simulink model "Steering"  (R2017a)
settings: Solver=VariableStepAuto  StartTime=0.0  StopTime=10  FixedStep=0.05  RelTol=1e-3
values from neighbouring files (symbols this model uses):
  distance_of_CG = vehical_length/2    (= 0.1825)    [initialize.m]
  H = Center_G(1)    [initialize.m]
  K = Center_G(2)    [initialize.m]
  psi_init = deg2rad(60)    [initialize.m]
  test_case = 2    [initialize.m]
  x0 = 0    [initialize.m]
  x_init = 0    [initialize.m]
  y0 = 0    [initialize.m]
  y_init = 1    [initialize.m]
undefined symbols (not defined in the file): parabora_coefficient, Radius, Theta, vehical_length, x_intersept, y_intersept
libraries: simulink_extras x5, frdmtfcshieldlib x2, simulink x1
settings Model: SnapshotInterval=1  Creator=dell  LastModifiedBy=dell
settings DebuggingCC: InheritedTsInSrcMsg=error

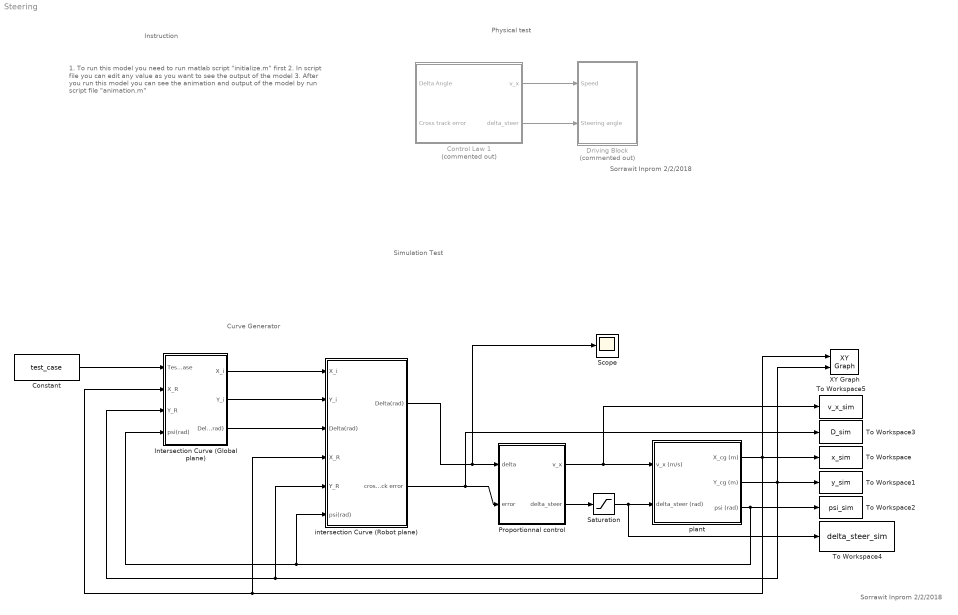
== system Steering ==
  note: Sorrawit Inprom
      | 2/2/2018
  note: Curve Generator
  note: Simulation Test
  note: Physical test
  note: Sorrawit Inprom
      | 2/2/2018
  note: Instruction
  note: 1. To run this model you need to run matlab script "initialize.m" first
      |
      | 2. In script file you can edit any value as you want to see the output of the model
      |
      | 3. After you run this model you can see the animation and output of the model by run script file "animation.m"
  Constant : Constant  Value=test_case
  Control Law 1 : Subsystem  Commented=on
  Driving Block : Subsystem  Commented=on
  Intersection Curve (Global plane) : Subsystem
  Proportionnal control : Subsystem
  Saturation : Saturate  UpperLimit=deg2rad(25)  LowerLimit=-deg2rad(25)
  Scope : Scope
  To Workspace : ToWorkspace  VariableName=x_sim  SaveFormat=Timeseries  SampleTime=-1
  To Workspace1 : ToWorkspace  VariableName=y_sim  SaveFormat=Timeseries  SampleTime=-1
  To Workspace2 : ToWorkspace  VariableName=psi_sim  SaveFormat=Timeseries  SampleTime=-1
  To Workspace3 : ToWorkspace  VariableName=D_sim  SaveFormat=Timeseries  SampleTime=-1
  To Workspace4 : ToWorkspace  VariableName=delta_steer_sim  SaveFormat=Timeseries  SampleTime=-1
  To Workspace5 : ToWorkspace  VariableName=v_x_sim  SaveFormat=Timeseries  SampleTime=-1
  XY Graph : simulink/Sinks/XY Graph  xmin=-5  xmax=5  ymin=-5  ymax=5  st=-1
  intersection Curve (Robot plane) : Subsystem
  plant : Subsystem  mask{vehicle_length=vehical_length, distance_of_CG=distance_of_CG}
      mask prompts: vehicle_length "length"; distance_of_CG "CG"
  wires:
  plant/1(X_cg (m)) -> XY Graph/1, To Workspace/1, intersection Curve (Robot plane)/4(X_R), Intersection Curve (Global plane)/2(X_R)
  plant/2(Y_cg (m)) -> XY Graph/2, To Workspace1/1, intersection Curve (Robot plane)/5(Y_R), Intersection Curve (Global plane)/3(Y_R)
  intersection Curve (Robot plane)/2(cross track error) -> To Workspace3/1, Proportionnal control/2(error)
  Proportionnal control/1(v_x) -> To Workspace5/1, plant/1(v_x (m/s))
  plant/3(psi (rad)) -> intersection Curve (Robot plane)/6(psi(rad)), Intersection Curve (Global plane)/4(psi(rad)), To Workspace2/1
  Constant/1 -> Intersection Curve (Global plane)/1(Test case)
  Intersection Curve (Global plane)/1("X_i ") -> intersection Curve (Robot plane)/1(X_i)
  Intersection Curve (Global plane)/2(Y_i) -> intersection Curve (Robot plane)/2(Y_i)
  Intersection Curve (Global plane)/3(Delta(rad)) -> intersection Curve (Robot plane)/3(Delta(rad))
  Saturation/1 -> To Workspace4/1, plant/2(delta_steer (rad))
  Proportionnal control/2(delta_steer) -> Saturation/1
  intersection Curve (Robot plane)/1("Delta(rad) ") -> Scope/1, Proportionnal control/1(delta)
  Control Law 1/1(v_x) -> Driving Block/1(Speed)
  Control Law 1/2(delta_steer) -> Driving Block/2(Steering angle)

== system Steering/Control Law 1 ==
  Delta Angle : Inport
  Cross track error : Inport  Port=2
  Abs : Abs
  Constant : Constant  Value=2
  Constant1 : Constant  Commented=on  Value=[0 ; 0]
  Divide : Product  Inputs=/
  Kp : Gain  Gain=5
  Kv : Gain
  Multiport Switch : MultiPortSwitch  Commented=on  DataPortOrder=Zero-based contiguous  Inputs=2  DataPortForDefault=Additional data port
  Sum : Sum  Inputs=|++
  Sum1 : Sum  Inputs=|++
  v_x : Outport  SampleTime=0.05
  delta_steer : Outport  Port=2  SampleTime=0.05
  wires:
  Constant/1 -> Sum/2
  Sum/1 -> Divide/1
  Constant1/1 -> Multiport Switch/2
  Divide/1 -> v_x/1
  Abs/1 -> Kv/1
  Kv/1 -> Sum/1
  Kp/1 -> delta_steer/1
  Delta Angle/1 -> Sum1/2
  Cross track error/1 -> Sum1/1, Abs/1
  Sum1/1 -> Kp/1

== system Steering/Driving Block ==
  Speed : Inport
  Steering angle : Inport  Port=2
  DC Motor : frdmtfcshieldlib/DC Motor  WhichMotor=A
      settings: SourceProductName=Simulink Coder Support Package for NXP FRDM-KL25Z Board  SourceProductBaseCode=EC_FREEDOM_BOARD
  Radians to Degrees1 : simulink_extras/Transformations/Radians to Degrees
  Saturation1 : Saturate  UpperLimit=20  LowerLimit=-20
  Servo Write : frdmtfcshieldlib/Servo Write  WhichServo=0  minAngle=-20.0  maxAngle=20.0
      settings: SourceProductName=Simulink Coder Support Package for NXP FRDM-KL25Z Board  SourceProductBaseCode=EC_FREEDOM_BOARD
  wires:
  Radians to Degrees1/1 -> Saturation1/1
  Saturation1/1 -> Servo Write/1
  Steering angle/1 -> Radians to Degrees1/1
  Speed/1 -> DC Motor/1

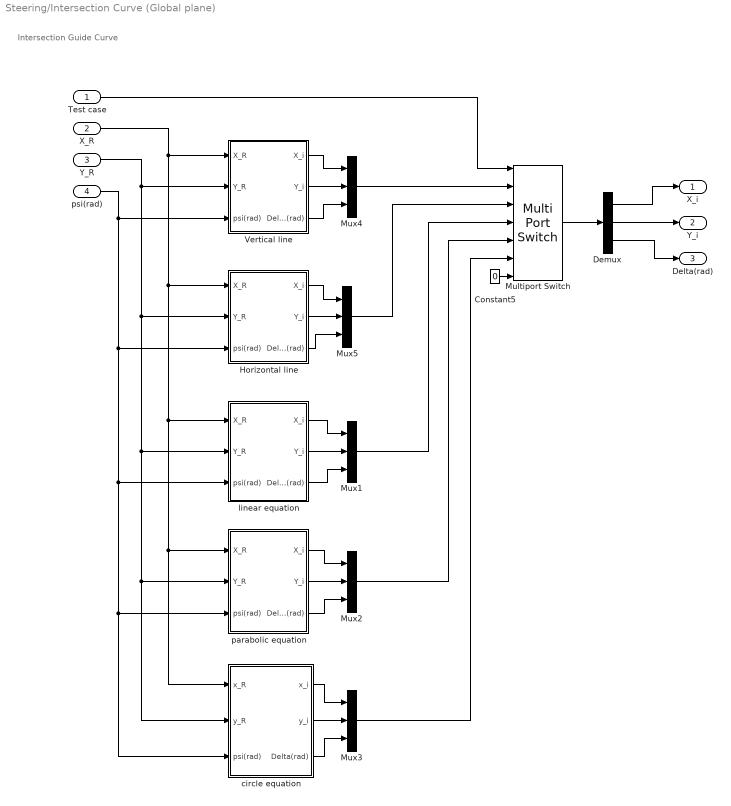
== system Steering/Intersection Curve (Global plane) ==
  note: Intersection Guide Curve
  Test case : Inport
  X_R : Inport  Port=2
  Y_R : Inport  Port=3
  psi(rad) : Inport  Port=4
  Constant5 : Constant  Value=0
  Demux : Demux  Outputs=3
  "Horizontal line " : Subsystem  mask{C=y_intersept}
      mask prompts: C "Y="
  Multiport Switch : MultiPortSwitch  DataPortOrder=Zero-based contiguous  Inputs=5  DataPortForDefault=Additional data port  DiagnosticForDefault=None
  Mux{1..5} (5 alike) : Mux  Inputs=3
  "Vertical line " : Subsystem  mask{C=x_intersept}
      mask prompts: C "X="
  circle equation : Subsystem  mask{H=H, K=K, r=Radius}
      mask prompts: H "Center_X"; K "Center_Y"; r "Radius"
  linear equation : Subsystem  mask{x0=x0, y0=y0, theta=Theta}
      mask prompts: theta "Theta(deg)"
  parabolic equation : Subsystem  mask{a=parabora_coefficient}
      mask prompts: a "Parabola characteristic"
  "X_i " : Outport
  Y_i : Outport  Port=2
  Delta(rad) : Outport  Port=3
  wires:
  psi(rad)/1 -> circle equation/3(psi(rad)), parabolic equation/3(psi(rad)), linear equation/3(psi(rad)), "Horizontal line "/3(psi(rad)), "Vertical line "/3(psi(rad))
  Y_R/1 -> circle equation/2(y_R), parabolic equation/2(Y_R), linear equation/2(Y_R), "Horizontal line "/2(Y_R), "Vertical line "/2(Y_R)
  Test case/1 -> Multiport Switch/1
  linear equation/3("Delta(rad) ") -> Mux1/3
  linear equation/1(X_i) -> Mux1/1
  Demux/2 -> Y_i/1
  Demux/1 -> "X_i "/1
  X_R/1 -> circle equation/1(x_R), parabolic equation/1(X_R), linear equation/1(X_R), "Horizontal line "/1(X_R), "Vertical line "/1(X_R)
  Multiport Switch/1 -> Demux/1
  Demux/3 -> Delta(rad)/1
  parabolic equation/1(X_i) -> Mux2/1
  parabolic equation/2(Y_i) -> Mux2/2
  parabolic equation/3("Delta(rad) ") -> Mux2/3
  linear equation/2(Y_i) -> Mux1/2
  circle equation/2(y_i) -> Mux3/2
  circle equation/1(x_i) -> Mux3/1
  circle equation/3(Delta(rad)) -> Mux3/3
  Constant5/1 -> Multiport Switch/7
  Mux1/1 -> Multiport Switch/4
  Mux2/1 -> Multiport Switch/5
  Mux3/1 -> Multiport Switch/6
  "Vertical line "/2(Y_i) -> Mux4/2
  "Vertical line "/1(X_i) -> Mux4/1
  "Vertical line "/3(Delta(rad)) -> Mux4/3
  "Horizontal line "/2(Y_i) -> Mux5/2
  "Horizontal line "/1(X_i) -> Mux5/1
  "Horizontal line "/3(Delta(rad)) -> Mux5/3
  Mux4/1 -> Multiport Switch/2
  Mux5/1 -> Multiport Switch/3

== system Steering/Proportionnal control ==
  delta : Inport
  error : Inport  Port=2
  Abs : Abs
  Constant : Constant  Value=0.5
  Constant1 : Constant  Commented=on  Value=[0 ; 0]
  Divide : Product  Inputs=/
  Kp : Gain  Gain=5
  Kv : Gain
  Multiport Switch : MultiPortSwitch  Commented=on  DataPortOrder=Zero-based contiguous  Inputs=2  DataPortForDefault=Additional data port
  Sum : Sum  Inputs=|++
  Sum1 : Sum  Inputs=|++
  v_x : Outport  SampleTime=0.1
  delta_steer : Outport  Port=2  SampleTime=0.05
  wires:
  Constant/1 -> Sum/2
  Sum/1 -> Divide/1
  Constant1/1 -> Multiport Switch/2
  Divide/1 -> v_x/1
  Abs/1 -> Kv/1
  Kv/1 -> Sum/1
  Kp/1 -> delta_steer/1
  delta/1 -> Sum1/2
  error/1 -> Sum1/1, Abs/1
  Sum1/1 -> Kp/1

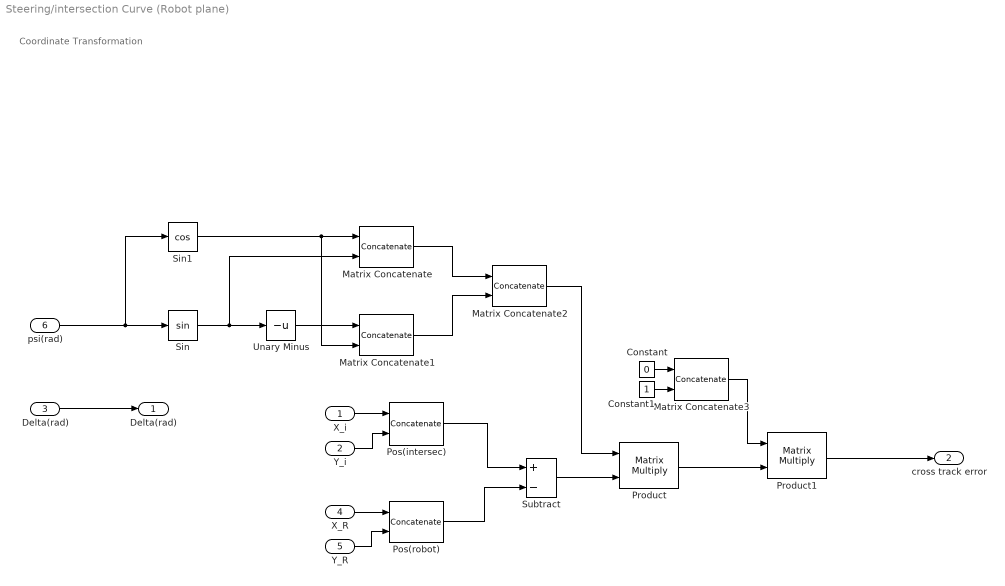
== system Steering/intersection Curve (Robot plane) ==
  note: Coordinate Transformation
  X_i : Inport
  Y_i : Inport  Port=2
  Delta(rad) : Inport  Port=3
  X_R : Inport  Port=4
  Y_R : Inport  Port=5
  psi(rad) : Inport  Port=6
  Constant : Constant  Value=0
  Constant1 : Constant
  Matrix Concatenate : Concatenate  Mode=Multidimensional array  ConcatenateDimension=2
  Matrix Concatenate1 : Concatenate  Mode=Multidimensional array  ConcatenateDimension=2
  Matrix Concatenate2 : Concatenate  Mode=Multidimensional array
  Matrix Concatenate3 : Concatenate  Mode=Multidimensional array  ConcatenateDimension=2
  "Pos(intersec) " : Concatenate  Mode=Multidimensional array
  Pos(robot) : Concatenate  Mode=Multidimensional array
  Product : Product  Multiplication=Matrix(*)
  Product1 : Product  Multiplication=Matrix(*)
  Sin : Trigonometry
  Sin1 : Trigonometry  Operator=cos
  Subtract : Sum  Inputs=+-
  Unary Minus : UnaryMinus
  "Delta(rad) " : Outport
  cross track error : Outport  Port=2
  wires:
  psi(rad)/1 -> Sin1/1, Sin/1
  Matrix Concatenate2/1 -> Product/1
  X_i/1 -> "Pos(intersec) "/1
  Y_i/1 -> "Pos(intersec) "/2
  Subtract/1 -> Product/2
  "Pos(intersec) "/1 -> Subtract/1
  Pos(robot)/1 -> Subtract/2
  Unary Minus/1 -> Matrix Concatenate1/1
  Y_R/1 -> Pos(robot)/2
  X_R/1 -> Pos(robot)/1
  Matrix Concatenate1/1 -> Matrix Concatenate2/2
  Sin1/1 -> Matrix Concatenate/1, Matrix Concatenate1/2
  Matrix Concatenate/1 -> Matrix Concatenate2/1
  Sin/1 -> Matrix Concatenate/2, Unary Minus/1
  Delta(rad)/1 -> "Delta(rad) "/1
  Product/1 -> Product1/2
  Constant/1 -> Matrix Concatenate3/1
  Constant1/1 -> Matrix Concatenate3/2
  Matrix Concatenate3/1 -> Product1/1
  Product1/1 -> cross track error/1

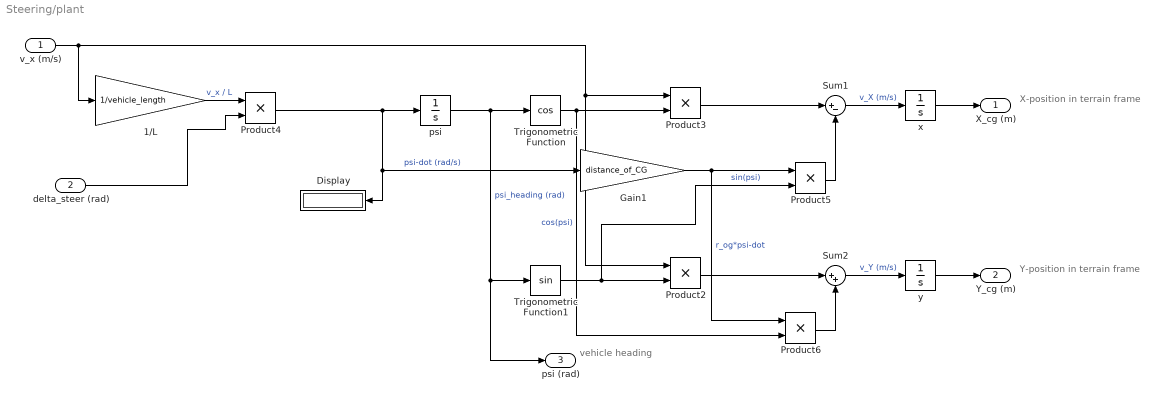
== system Steering/plant ==
  note: vehicle
      | heading
  note: X-position in
      | terrain frame
  note: Y-position in
      | terrain frame
  v_x (m/s) : Inport
  delta_steer (rad) : Inport  Port=2
  1/L : Gain  Gain=1/vehicle_length
  Display : Display
  Gain1 : Gain  Gain=distance_of_CG
  Product{2..6} (5 alike) : Product  RndMeth=Zero
  Sum1 : Sum  Inputs=|+-
  Sum2 : Sum  Inputs=|++
  Trigonometric Function : Trigonometry  Operator=cos
  Trigonometric Function1 : Trigonometry
  psi : Integrator  InitialCondition=psi_init
  x : Integrator  InitialCondition=x_init
  y : Integrator  InitialCondition=y_init
  X_cg (m) : Outport
  Y_cg (m) : Outport  Port=2
  psi (rad) : Outport  Port=3
  wires:
  psi/1 -> Trigonometric Function/1, psi (rad)/1, Trigonometric Function1/1  "psi_heading (rad)"
  x/1 -> X_cg (m)/1
  Trigonometric Function/1 -> Product6/2, Product3/2  "cos(psi)"
  Product4/1 -> Gain1/1, Display/1, psi/1  "psi-dot (rad/s)"
  Sum2/1 -> y/1  "v_Y (m/s)"
  Product6/1 -> Sum2/2
  Product3/1 -> Sum1/1
  y/1 -> Y_cg (m)/1
  Trigonometric Function1/1 -> Product2/2, Product5/2  "sin(psi)"
  Gain1/1 -> Product5/1, Product6/1  "r_og*psi-dot"
  1/L/1 -> Product4/1  "v_x / L"
  Product2/1 -> Sum2/1
  v_x (m/s)/1 -> Product2/1, Product3/1, 1/L/1
  Product5/1 -> Sum1/2
  Sum1/1 -> x/1  "v_X (m/s)"
  delta_steer (rad)/1 -> Product4/2

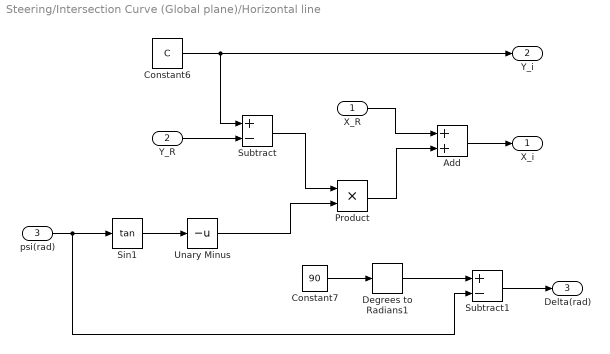
== system Steering/Intersection Curve (Global plane)/Horizontal line  ==
  X_R : Inport
  Y_R : Inport  Port=2
  psi(rad) : Inport  Port=3
  Add : Sum
  Constant6 : Constant  Value=C
  Constant7 : Constant  Value=90
  Degrees to Radians1 : simulink_extras/Transformations/Degrees to Radians
  Product : Product
  Sin1 : Trigonometry  Operator=tan
  Subtract : Sum  Inputs=+-
  Subtract1 : Sum  Inputs=+-
  Unary Minus : UnaryMinus
  X_i : Outport
  Y_i : Outport  Port=2
  Delta(rad) : Outport  Port=3
  wires:
  psi(rad)/1 -> Subtract1/2, Sin1/1
  Constant6/1 -> Y_i/1, Subtract/1
  Constant7/1 -> Degrees to Radians1/1
  Degrees to Radians1/1 -> Subtract1/1
  Subtract1/1 -> Delta(rad)/1
  Y_R/1 -> Subtract/2
  Sin1/1 -> Unary Minus/1
  Subtract/1 -> Product/1
  Unary Minus/1 -> Product/2
  X_R/1 -> Add/1
  Product/1 -> Add/2
  Add/1 -> X_i/1

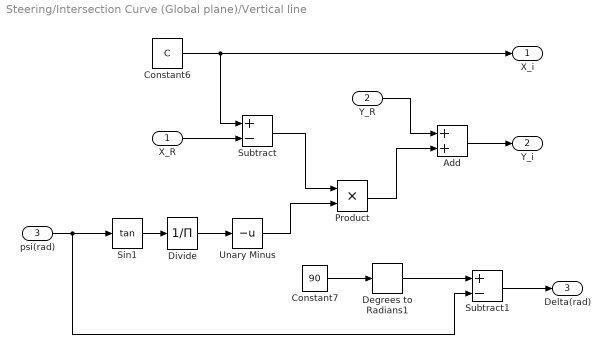
== system Steering/Intersection Curve (Global plane)/Vertical line  ==
  X_R : Inport
  Y_R : Inport  Port=2
  psi(rad) : Inport  Port=3
  Add : Sum
  Constant6 : Constant  Value=C
  Constant7 : Constant  Value=90
  Degrees to Radians1 : simulink_extras/Transformations/Degrees to Radians
  Divide : Product  Inputs=/
  Product : Product
  Sin1 : Trigonometry  Operator=tan
  Subtract : Sum  Inputs=+-
  Subtract1 : Sum  Inputs=+-
  Unary Minus : UnaryMinus
  X_i : Outport
  Y_i : Outport  Port=2
  Delta(rad) : Outport  Port=3
  wires:
  psi(rad)/1 -> Subtract1/2, Sin1/1
  Constant6/1 -> Subtract/1, X_i/1
  Constant7/1 -> Degrees to Radians1/1
  Degrees to Radians1/1 -> Subtract1/1
  Subtract1/1 -> Delta(rad)/1
  Subtract/1 -> Product/1
  Unary Minus/1 -> Product/2
  Product/1 -> Add/2
  X_R/1 -> Subtract/2
  Y_R/1 -> Add/1
  Sin1/1 -> Divide/1
  Divide/1 -> Unary Minus/1
  Add/1 -> Y_i/1

== system Steering/Intersection Curve (Global plane)/circle equation ==
  x_R : Inport
  y_R : Inport  Port=2
  psi(rad) : Inport  Port=3
  Select solution : Subsystem
  find intersection : Subsystem
  x_i : Outport
  y_i : Outport  Port=2
  Delta(rad) : Outport  Port=3
  wires:
  x_R/1 -> find intersection/1(X_R), Select solution/1(x_R)
  y_R/1 -> find intersection/2(Y_R), Select solution/2(y_R)
  psi(rad)/1 -> find intersection/3(psi(rad))
  find intersection/2(sol2) -> Select solution/4(sol2)
  find intersection/1(sol1) -> Select solution/3(sol1)
  Select solution/1(x_i) -> x_i/1
  Select solution/2(y_i) -> y_i/1
  find intersection/3(Delta(rad)) -> Delta(rad)/1

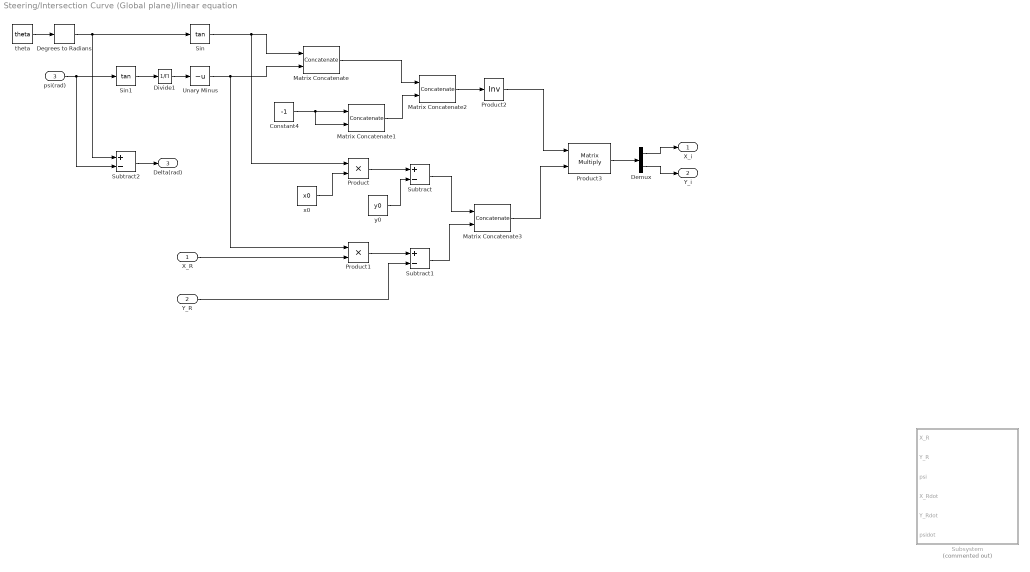
== system Steering/Intersection Curve (Global plane)/linear equation ==
  X_R : Inport
  Y_R : Inport  Port=2
  psi(rad) : Inport  Port=3
  Constant4 : Constant  Value=-1
  Degrees to Radians : simulink_extras/Transformations/Degrees to Radians
  Demux : Demux  Outputs=2
  Divide1 : Product  Inputs=/
  Matrix Concatenate : Concatenate  Mode=Multidimensional array
  Matrix Concatenate1 : Concatenate  Mode=Multidimensional array
  Matrix Concatenate2 : Concatenate  Mode=Multidimensional array  ConcatenateDimension=2
  Matrix Concatenate3 : Concatenate  Mode=Multidimensional array
  Product : Product
  Product1 : Product
  Product2 : Product  Inputs=/  Multiplication=Matrix(*)
  Product3 : Product  Multiplication=Matrix(*)
  Sin : Trigonometry  Operator=tan
  Sin1 : Trigonometry  Operator=tan
  Subsystem : Subsystem  Commented=on
  Subtract : Sum  Inputs=+-
  Subtract1 : Sum  Inputs=+-
  Subtract2 : Sum  Inputs=+-
  Unary Minus : UnaryMinus
  theta : Constant  Value=theta
  x0 : Constant  Value=x0
  y0 : Constant  Value=y0
  X_i : Outport
  Y_i : Outport  Port=2
  "Delta(rad) " : Outport  Port=3
  wires:
  Matrix Concatenate2/1 -> Product2/1
  X_R/1 -> Product1/2
  Demux/2 -> Y_i/1
  Matrix Concatenate3/1 -> Product3/2
  Divide1/1 -> Unary Minus/1
  Sin1/1 -> Divide1/1
  y0/1 -> Subtract/2
  x0/1 -> Product/2
  Demux/1 -> X_i/1
  Unary Minus/1 -> Product1/1, Matrix Concatenate/2
  Subtract/1 -> Matrix Concatenate3/1
  Y_R/1 -> Subtract1/2
  Product/1 -> Subtract/1
  Product1/1 -> Subtract1/1
  Subtract1/1 -> Matrix Concatenate3/2
  psi(rad)/1 -> Sin1/1, Subtract2/2
  Constant4/1 -> Matrix Concatenate1/2, Matrix Concatenate1/1
  Matrix Concatenate1/1 -> Matrix Concatenate2/2
  Product2/1 -> Product3/1
  Sin/1 -> Product/1, Matrix Concatenate/1
  theta/1 -> Degrees to Radians/1
  Product3/1 -> Demux/1
  Subtract2/1 -> "Delta(rad) "/1
  Matrix Concatenate/1 -> Matrix Concatenate2/1
  Degrees to Radians/1 -> Sin/1, Subtract2/1

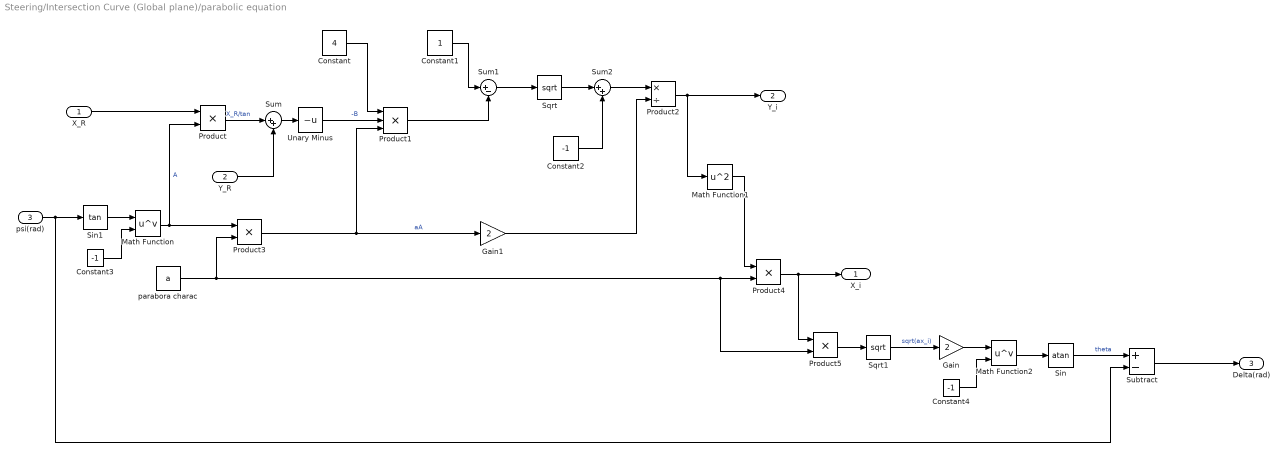
== system Steering/Intersection Curve (Global plane)/parabolic equation ==
  X_R : Inport
  Y_R : Inport  Port=2
  psi(rad) : Inport  Port=3
  Constant : Constant  Value=4
  Constant1 : Constant
  Constant2 : Constant  Value=-1
  Constant3 : Constant  Value=-1
  Constant4 : Constant  Value=-1
  Gain : Gain  Gain=2
  Gain1 : Gain  Gain=2
  Math Function : Math  Operator=pow  SaturateOnIntegerOverflow=on
  Math Function1 : Math  Operator=square  SaturateOnIntegerOverflow=on
  Math Function2 : Math  Operator=pow  SaturateOnIntegerOverflow=on
  Product{,3..5} (4 alike) : Product
  Product1 : Product  Inputs=3
  Product2 : Product  Inputs=*/
  Sin : Trigonometry  Operator=atan
  Sin1 : Trigonometry  Operator=tan
  Sqrt : Sqrt  SaturateOnIntegerOverflow=on
  Sqrt1 : Sqrt  SaturateOnIntegerOverflow=on
  Subtract : Sum  Inputs=+-
  Sum : Sum  Inputs=|++
  Sum1 : Sum  Inputs=|+-
  Sum2 : Sum  Inputs=|++
  Unary Minus : UnaryMinus
  parabora charac : Constant  Value=a
  X_i : Outport
  Y_i : Outport  Port=2
  "Delta(rad) " : Outport  Port=3
  wires:
  parabora charac/1 -> Product5/2, Product4/2, Product3/2
  Math Function1/1 -> Product4/1
  Product4/1 -> Product5/1, X_i/1
  X_R/1 -> Product/1
  Sqrt/1 -> Sum2/1
  Product2/1 -> Y_i/1, Math Function1/1
  Gain1/1 -> Product2/2
  Constant1/1 -> Sum1/1
  Constant2/1 -> Sum2/2
  Product/1 -> Sum/1  "X_R/tan"
  Sum/1 -> Unary Minus/1
  Unary Minus/1 -> Product1/2  "-B"
  Y_R/1 -> Sum/2
  Product3/1 -> Gain1/1, Product1/3  "aA"
  Sum1/1 -> Sqrt/1
  Product1/1 -> Sum1/2
  Constant/1 -> Product1/1
  Sum2/1 -> Product2/1
  Sin1/1 -> Math Function/1
  psi(rad)/1 -> Subtract/2, Sin1/1
  Constant3/1 -> Math Function/2
  Math Function/1 -> Product3/1, Product/2  "A"
  Product5/1 -> Sqrt1/1
  Sqrt1/1 -> Gain/1  "sqrt(ax_i)"
  Gain/1 -> Math Function2/1
  Constant4/1 -> Math Function2/2
  Math Function2/1 -> Sin/1
  Sin/1 -> Subtract/1  "theta"
  Subtract/1 -> "Delta(rad) "/1

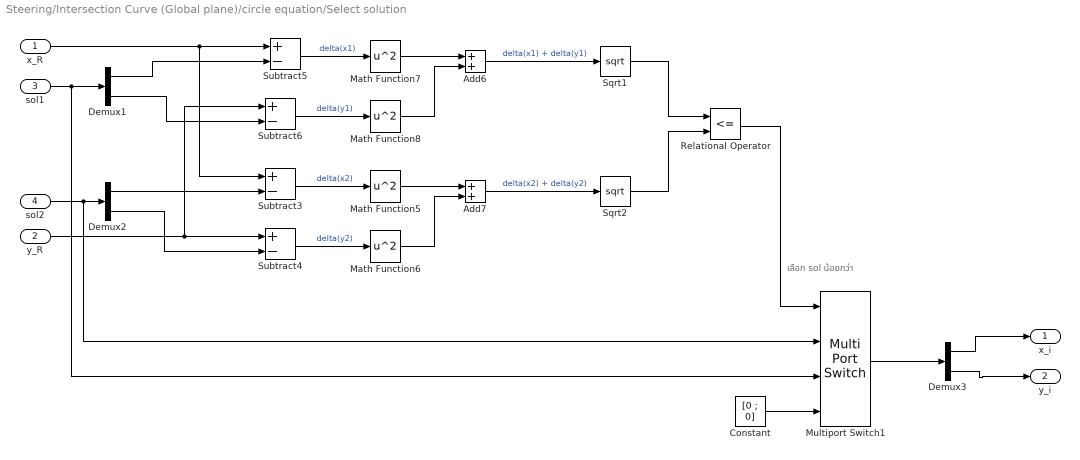
== system Steering/Intersection Curve (Global plane)/circle equation/Select solution ==
  note: เลือก sol น้อยกว่า
  x_R : Inport
  y_R : Inport  Port=2
  sol1 : Inport  Port=3
  sol2 : Inport  Port=4
  Add6 : Sum
  Add7 : Sum
  Constant : Constant  Value=[0 ; 0]
  Demux1 : Demux  Outputs=2
  Demux2 : Demux  Outputs=2
  Demux3 : Demux  Outputs=2
  Math Function{5..8} (4 alike) : Math  Operator=square  SaturateOnIntegerOverflow=on
  Multiport Switch1 : MultiPortSwitch  DataPortOrder=Zero-based contiguous  Inputs=2  DataPortForDefault=Additional data port  DiagnosticForDefault=None
  Relational Operator : RelationalOperator  Operator=<=  OutDataTypeStr=boolean  RndMeth=Simplest
  Sqrt1 : Sqrt  SaturateOnIntegerOverflow=on
  Sqrt2 : Sqrt  SaturateOnIntegerOverflow=on
  Subtract{3..6} (4 alike) : Sum  Inputs=+-
  x_i : Outport
  y_i : Outport  Port=2
  wires:
  Demux1/2 -> Subtract6/2
  Subtract3/1 -> Math Function5/1  "delta(x2)"
  Math Function8/1 -> Add6/2
  Demux2/2 -> Subtract4/2
  Demux2/1 -> Subtract3/2
  Subtract5/1 -> Math Function7/1  "delta(x1)"
  Subtract6/1 -> Math Function8/1  "delta(y1)"
  Sqrt2/1 -> Relational Operator/2
  Add7/1 -> Sqrt2/1  "delta(x2) + delta(y2)"
  Add6/1 -> Sqrt1/1  "delta(x1) + delta(y1)"
  Math Function6/1 -> Add7/2
  Math Function7/1 -> Add6/1
  Relational Operator/1 -> Multiport Switch1/1
  Sqrt1/1 -> Relational Operator/1
  Subtract4/1 -> Math Function6/1  "delta(y2)"
  Demux1/1 -> Subtract5/2
  sol1/1 -> Multiport Switch1/3, Demux1/1
  y_R/1 -> Subtract6/1, Subtract4/1
  sol2/1 -> Multiport Switch1/2, Demux2/1
  x_R/1 -> Subtract3/1, Subtract5/1
  Multiport Switch1/1 -> Demux3/1
  Math Function5/1 -> Add7/1
  Demux3/2 -> y_i/1
  Constant/1 -> Multiport Switch1/4
  Demux3/1 -> x_i/1

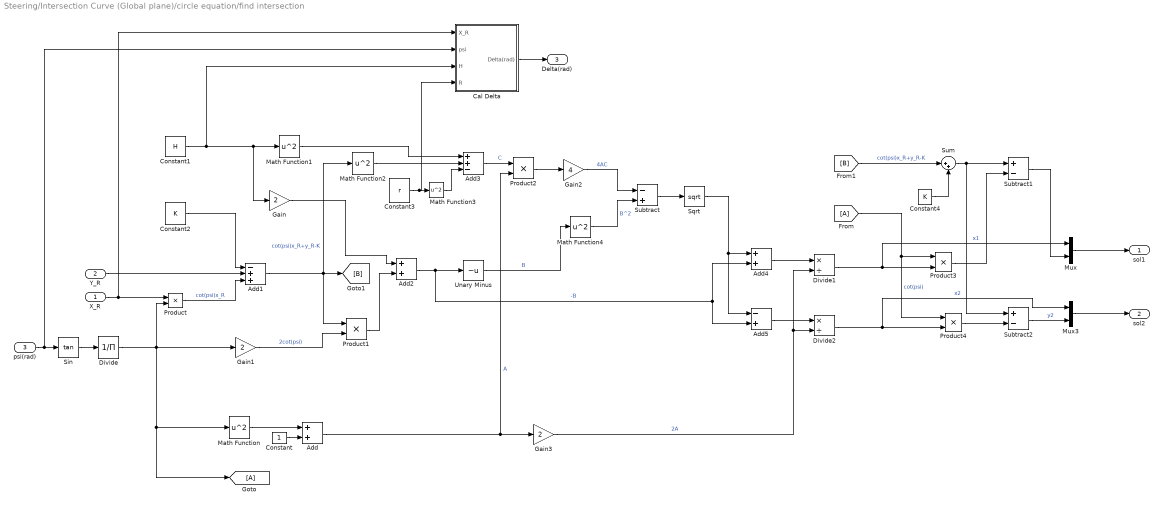
== system Steering/Intersection Curve (Global plane)/circle equation/find intersection ==
  X_R : Inport
  Y_R : Inport  Port=2
  psi(rad) : Inport  Port=3
  Add : Sum
  Add1 : Sum  Inputs=-++
  Add2 : Sum
  Add3 : Sum  Inputs=++-
  Add4 : Sum
  Add5 : Sum  Inputs=-+
  Cal Delta : Subsystem
  Constant : Constant
  Constant1 : Constant  Value=H
  Constant2 : Constant  Value=K
  Constant3 : Constant  Value=r
  Constant4 : Constant  Value=K
  Divide : Product  Inputs=/
  Divide1 : Product  Inputs=*/
  Divide2 : Product  Inputs=*/
  Gain : Gain  Gain=2
  Gain1 : Gain  Gain=2
  Gain2 : Gain  Gain=4
  Gain3 : Gain  Gain=2
  Math Function{,1..4} (5 alike) : Math  Operator=square  SaturateOnIntegerOverflow=on
  Mux : Mux  Inputs=2
  Mux3 : Mux  Inputs=2
  Product{,1..4} (5 alike) : Product
  Sin : Trigonometry  Operator=tan
  Sqrt : Sqrt  SaturateOnIntegerOverflow=on
  Subtract : Sum  Inputs=-+
  Subtract1 : Sum  Inputs=+-
  Subtract2 : Sum  Inputs=+-
  Sum : Sum  Inputs=|++
  Unary Minus : UnaryMinus
  sol1 : Outport
  sol2 : Outport  Port=2
  Delta(rad) : Outport  Port=3
  wires:
  Mux3/1 -> sol2/1
  Mux/1 -> sol1/1
  Subtract1/1 -> Mux/2
  Subtract2/1 -> Mux3/2  "y2"
  [B] -> Sum/1  "cot(psi)x_R+y_R-K"
  Product2/1 -> Gain2/1
  Product4/1 -> Subtract2/2
  Constant3/1 -> Cal Delta/4(R), Math Function3/1
  Sum/1 -> Subtract2/1, Subtract1/1
  Divide/1 -> Gain1/1, Math Function/1, [A], Product/2
  Math Function2/1 -> Add3/2
  Math Function1/1 -> Add3/1
  Unary Minus/1 -> Math Function4/1  "B"
  [A] -> Product4/1, Product3/1  "cot(psi)"
  Subtract/1 -> Sqrt/1
  Gain2/1 -> Subtract/1  "4AC"
  Constant4/1 -> Sum/2
  Sqrt/1 -> Add5/1, Add4/1
  Add2/1 -> Add5/2, Add4/2, Unary Minus/1  "-B"
  Product3/1 -> Subtract1/2
  Y_R/1 -> Add1/2
  Constant1/1 -> Cal Delta/3(H), Gain/1, Math Function1/1
  Add/1 -> Gain3/1, Product2/2  "A"
  Constant/1 -> Add/2
  Product1/1 -> Add2/2
  Math Function/1 -> Add/1
  Gain3/1 -> Divide1/2, Divide2/2  "2A"
  Divide1/1 -> Mux/1, Product3/2  "x1"
  Divide2/1 -> Mux3/1, Product4/2  "x2"
  Product/1 -> Add1/3  "cot(psi)x_R"
  psi(rad)/1 -> Cal Delta/2("psi "), Sin/1
  Sin/1 -> Divide/1
  Add1/1 -> [B], Math Function2/1, Product1/1  "cot(psi)x_R+y_R-K"
  Math Function3/1 -> Add3/3
  Constant2/1 -> Add1/1
  Add5/1 -> Divide2/1
  Add3/1 -> Product2/1  "C"
  Gain/1 -> Add2/1
  Add4/1 -> Divide1/1
  X_R/1 -> Cal Delta/1(X_R), Product/1
  Gain1/1 -> Product1/2  "2cot(psi)"
  Math Function4/1 -> Subtract/2  "B^2"
  Cal Delta/1(Delta(rad)) -> Delta(rad)/1

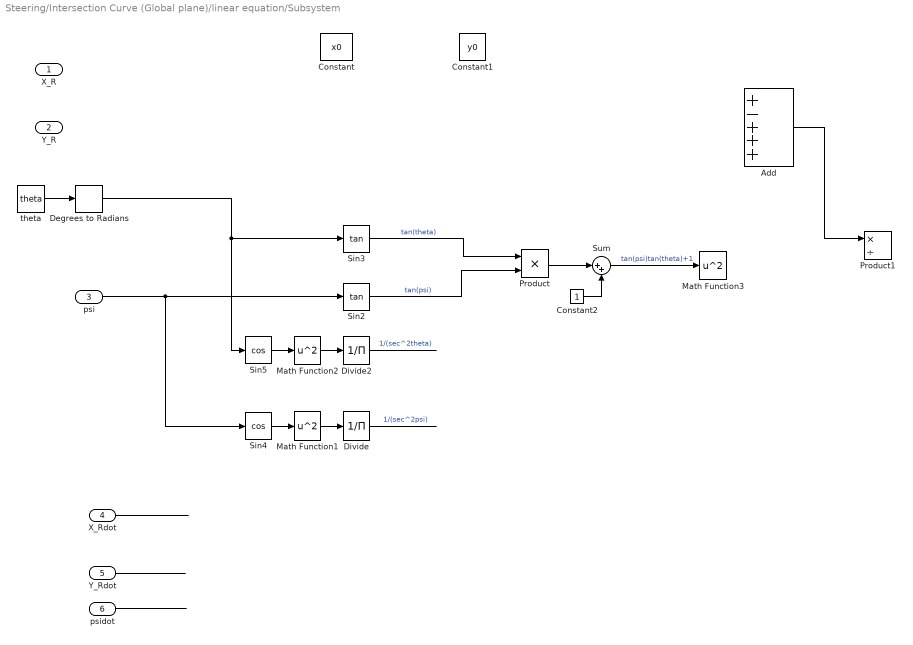
== system Steering/Intersection Curve (Global plane)/linear equation/Subsystem ==
  X_R : Inport
  "Y_R " : Inport  Port=2
  psi : Inport  Port=3
  X_Rdot : Inport  Port=4
  Y_Rdot : Inport  Port=5
  psidot : Inport  Port=6
  Add : Sum  Inputs=+-+++
  Constant : Constant  Value=x0
  Constant1 : Constant  Value=y0
  Constant2 : Constant
  Degrees to Radians : simulink_extras/Transformations/Degrees to Radians
  Divide : Product  Inputs=/
  Divide2 : Product  Inputs=/
  Math Function1 : Math  Operator=square  SaturateOnIntegerOverflow=on
  Math Function2 : Math  Operator=square  SaturateOnIntegerOverflow=on
  Math Function3 : Math  Operator=square  SaturateOnIntegerOverflow=on
  Product : Product
  Product1 : Product  Inputs=*/
  Sin2 : Trigonometry  Operator=tan
  Sin3 : Trigonometry  Operator=tan
  Sin4 : Trigonometry  Operator=cos
  Sin5 : Trigonometry  Operator=cos
  Sum : Sum  Inputs=|++
  theta : Constant  Value=theta
  wires:
  Sin3/1 -> Product/1  "tan(theta)"
  Sin4/1 -> Math Function1/1
  Math Function1/1 -> Divide/1
  Divide/1 -> ?  "1/(sec^2psi)"
  X_Rdot/1 -> ?
  Y_Rdot/1 -> ?
  psidot/1 -> ?
  Math Function2/1 -> Divide2/1
  Sin5/1 -> Math Function2/1
  Divide2/1 -> ?  "1/(sec^2theta)"
  psi/1 -> Sin4/1, Sin2/1
  Sin2/1 -> Product/2  "tan(psi)"
  Degrees to Radians/1 -> Sin5/1, Sin3/1
  theta/1 -> Degrees to Radians/1
  Product/1 -> Sum/1
  Constant2/1 -> Sum/2
  Sum/1 -> Math Function3/1  "tan(psi)tan(theta)+1"
  Add/1 -> Product1/1

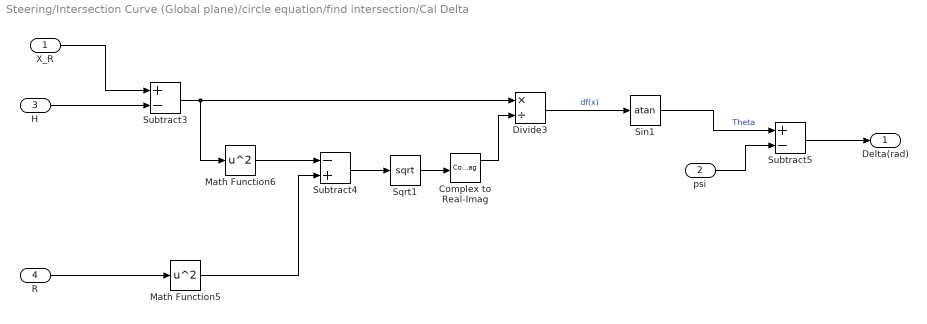
== system Steering/Intersection Curve (Global plane)/circle equation/find intersection/Cal Delta ==
  X_R : Inport
  "psi " : Inport  Port=2
  H : Inport  Port=3
  R : Inport  Port=4
  Complex to Real-Imag : ComplexToRealImag
  Divide3 : Product  Inputs=*/
  Math Function5 : Math  Operator=square  RndMeth=Zero  SaturateOnIntegerOverflow=on
  Math Function6 : Math  Operator=square  RndMeth=Zero  SaturateOnIntegerOverflow=on
  Sin1 : Trigonometry  Operator=atan
  Sqrt1 : Sqrt  SaturateOnIntegerOverflow=on
  Subtract3 : Sum  Inputs=+-
  Subtract4 : Sum  Inputs=-+
  Subtract5 : Sum  Inputs=+-
  Delta(rad) : Outport
  wires:
  Subtract3/1 -> Divide3/1, Math Function6/1
  Divide3/1 -> Sin1/1  "df(x)"
  "psi "/1 -> Subtract5/2
  H/1 -> Subtract3/2
  X_R/1 -> Subtract3/1
  Subtract4/1 -> Sqrt1/1
  Sin1/1 -> Subtract5/1  "Theta"
  Math Function6/1 -> Subtract4/1
  Math Function5/1 -> Subtract4/2
  R/1 -> Math Function5/1
  Subtract5/1 -> Delta(rad)/1
  Sqrt1/1 -> Complex to Real-Imag/1
  Complex to Real-Imag/1 -> Divide3/2
